simulink model "A2sim"  (R2022a)
settings: Solver=VariableStepAuto  StartTime=0.0  StopTime=10.0  RelTol=1e-3
undefined symbols (not defined in the file): ysp
settings Model: Creator=tanzc  LastModifiedBy=tanzc

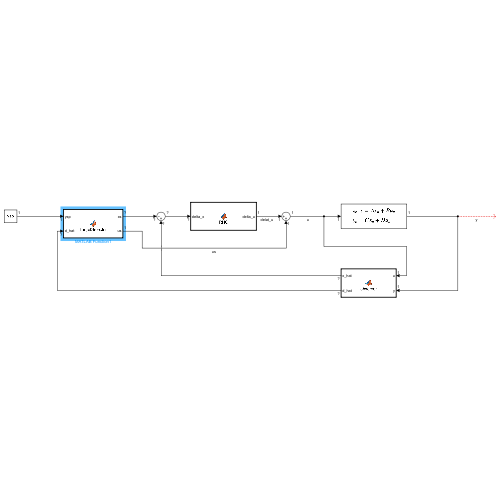
[thumbnail: Simulink's stored preview of the top-level diagram]
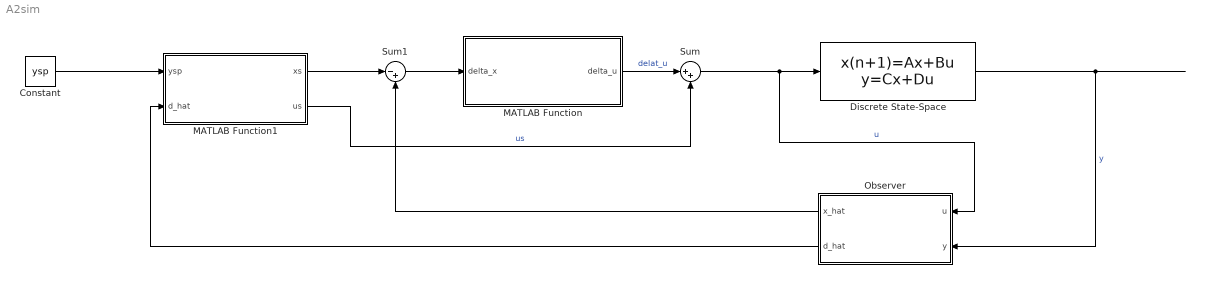
== system A2sim ==
  Constant : Constant  Value=ysp
  Discrete State-Space : DiscreteStateSpace  SampleTime=-1
  MATLAB Function : MATLAB Function  TreatAsAtomicUnit=on
  MATLAB Function1 : MATLAB Function  TreatAsAtomicUnit=on
  Observer : MATLAB Function  TreatAsAtomicUnit=on
  Sum : Sum  Inputs=|++
  Sum1 : Sum  Inputs=|-+
  wires:
  Discrete State-Space/1 -> Observer/2(y)  "y"
  Sum/1 -> Observer/1(u), Discrete State-Space/1  "u"
  Sum1/1 -> MATLAB Function/1(delta_x)
  MATLAB Function1/1(xs) -> Sum1/1
  Observer/1(x_hat) -> Sum1/2
  Observer/2(d_hat) -> MATLAB Function1/2(d_hat)
  Constant/1 -> MATLAB Function1/1(ysp)
  MATLAB Function1/2(us) -> Sum/2  "us"
  MATLAB Function/1(delta_u) -> Sum/1  "delat_u"

== matlab function A2sim/Observer ==
  data: u input; x_hat output; y input; d_hat output
function [x_hat, d_hat] = observer(u,y)

y = u;

== matlab function A2sim/MATLAB Function1 ==
  data: ysp input; xs output; d_hat input; us output
function [xs,us] = TargetSelector(ysp, d_hat)
    M = [eye(n)-A -B;
         H*C, zeros(size(H*C,1),m)];
    P = [Bd*d_hat;ysp-H*Cd];
    v = inv(M)*P;
    xs = v(1:n);
    us = v(n+1:end);

== matlab function A2sim/MATLAB Function ==
  data: delta_x input; delta_u output
function delta_u = RHC(delta_x)
